simulink model "SystemQ"  (R2014b)
settings: Solver=ode23  StartTime=0.0  StopTime=inf  RelTol=10e-3
PreLoadFcn:
  | initSysQ;
  | runSysQ;
undefined symbols (not defined in the file): Controllers, CR, dim, fdesignblkfcn, G, gcbh, lib, serial, Tjoint, Tpid, X, Y, Z
libraries: sm_lib x62, nesl_utility x28, simulink x10, roblocks x5, instrumentlib x2, dspmathops x1, dspinverses x1, dspmtrx3 x1
(part 3 of 3)

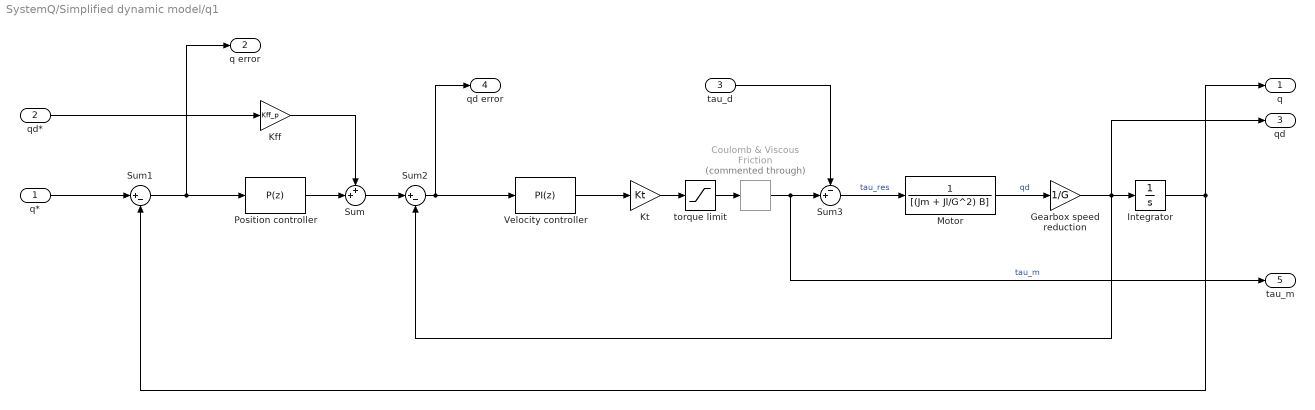
== system SystemQ/Simplified dynamic model/q1 ==
  q* : Inport
  qd* : Inport  Port=2
  tau_d : Inport  Port=3
  Coulomb & Viscous Friction : simulink/Discontinuities/Coulomb & Viscous Friction  Commented=through  offset=0.126  gain=1
  Gearbox speed reduction : Gain  Gain=1/G
  Integrator : Integrator
  Kff : Gain  Gain=Kff_p
  Kt : Gain  Gain=Kt
  Motor : TransferFcn  Denominator=[(Jm + Jl/G^2) B]  ContinuousStateAttributes='qd'
  Position controller : simulink/Continuous/PID Controller  Controller=P  TimeDomain=Discrete-time  SampleTime=Ts  IntegratorMethod=Forward Euler  FilterMethod=Forward Euler  Form=Parallel  P=Kp_p  I=Ki_p  D=Kd_p  N=100  InitialConditionSource=internal  InitialConditionForIntegrator=0  InitialConditionForFilter=0  ExternalReset=none  LimitOutput=off  UpperSaturationLimit=1  LowerSaturationLimit=-1  LinearizeAsGain=on  AntiWindupMode=none  Kb=1  TrackingMode=off  Kt=1  PParamMin=[]  PParamMax=[]  IParamMin=[]  IParamMax=[]  DParamMin=[]  DParamMax=[]  NParamMin=[]  NParamMax=[]  KbParamMin=[]  KbParamMax=[]  KtParamMin=[]  KtParamMax=[]  POutMin=[]  POutMax=[]  IOutMin=[]  IOutMax=[]  DOutMin=[]  DOutMax=[]  NOutMin=[]  NOutMax=[]  KbOutMin=[]  KbOutMax=[]  KtOutMin=[]  KtOutMax=[]  IntegratorOutMin=[]  IntegratorOutMax=[]  FilterOutMin=[]  FilterOutMax=[]  SumOutMin=[]  SumOutMax=[]  SumI1OutMin=[]  SumI1OutMax=[]  SumI2OutMin=[]  SumI2OutMax=[]  SumI3OutMin=[]  SumI3OutMax=[]  SumDOutMin=[]  SumDOutMax=[]  SaturationOutMin=[]  SaturationOutMax=[]  IntegratorContinuousStateAttributes=''  IntegratorStateMustResolveToSignalObject=off  IntegratorRTWStateStorageClass=Auto  FilterContinuousStateAttributes=''  FilterStateMustResolveToSignalObject=off  FilterRTWStateStorageClass=Auto  DifferentiatorICPrevScaledInput=0  DifferentiatorOutMin=[]  DifferentiatorOutMax=[]  UseFilter=on
  Sum : Sum  Inputs=++|
  Sum1 : Sum  Inputs=|+-
  Sum2 : Sum  Inputs=|+-
  Sum3 : Sum  Inputs=-+|
  Velocity controller : simulink/Continuous/PID Controller  Controller=PI  TimeDomain=Discrete-time  SampleTime=Ts  IntegratorMethod=Forward Euler  FilterMethod=Forward Euler  Form=Parallel  P=Kp_v  I=Ki_v  D=Kd_v  N=100  InitialConditionSource=internal  InitialConditionForIntegrator=0  InitialConditionForFilter=0  ExternalReset=none  LimitOutput=on  UpperSaturationLimit=4  LowerSaturationLimit=-4  LinearizeAsGain=on  AntiWindupMode=clamping  Kb=1  TrackingMode=off  Kt=1  PParamMin=[]  PParamMax=[]  IParamMin=[]  IParamMax=[]  DParamMin=[]  DParamMax=[]  NParamMin=[]  NParamMax=[]  KbParamMin=[]  KbParamMax=[]  KtParamMin=[]  KtParamMax=[]  POutMin=[]  POutMax=[]  IOutMin=[]  IOutMax=[]  DOutMin=[]  DOutMax=[]  NOutMin=[]  NOutMax=[]  KbOutMin=[]  KbOutMax=[]  KtOutMin=[]  KtOutMax=[]  IntegratorOutMin=[]  IntegratorOutMax=[]  FilterOutMin=[]  FilterOutMax=[]  SumOutMin=[]  SumOutMax=[]  SumI1OutMin=[]  SumI1OutMax=[]  SumI2OutMin=[]  SumI2OutMax=[]  SumI3OutMin=[]  SumI3OutMax=[]  SumDOutMin=[]  SumDOutMax=[]  SaturationOutMin=[]  SaturationOutMax=[]  IntegratorContinuousStateAttributes=''  IntegratorStateMustResolveToSignalObject=off  IntegratorRTWStateStorageClass=Auto  FilterContinuousStateAttributes=''  FilterStateMustResolveToSignalObject=off  FilterRTWStateStorageClass=Auto  DifferentiatorICPrevScaledInput=0  DifferentiatorOutMin=[]  DifferentiatorOutMax=[]  UseFilter=on
  torque limit : Saturate  UpperLimit=tau_max  LowerLimit=-tau_max
  q : Outport
  q error : Outport  Port=2
  qd : Outport  Port=3
  qd error : Outport  Port=4
  tau_m : Outport  Port=5
  wires:
  Sum1/1 -> Position controller/1, q error/1
  q*/1 -> Sum1/1
  Integrator/1 -> Sum1/2, q/1
  Sum/1 -> Sum2/1
  Sum3/1 -> Motor/1  "tau_res"
  Sum2/1 -> Velocity controller/1, qd error/1
  Motor/1 -> Gearbox speed reduction/1  "qd"
  tau_d/1 -> Sum3/1
  torque limit/1 -> Coulomb & Viscous Friction/1
  qd*/1 -> Kff/1
  Kt/1 -> torque limit/1
  Velocity controller/1 -> Kt/1
  Kff/1 -> Sum/1
  Position controller/1 -> Sum/2
  Coulomb & Viscous Friction/1 -> Sum3/2, tau_m/1  "tau_m"
  Gearbox speed reduction/1 -> Sum2/2, qd/1, Integrator/1

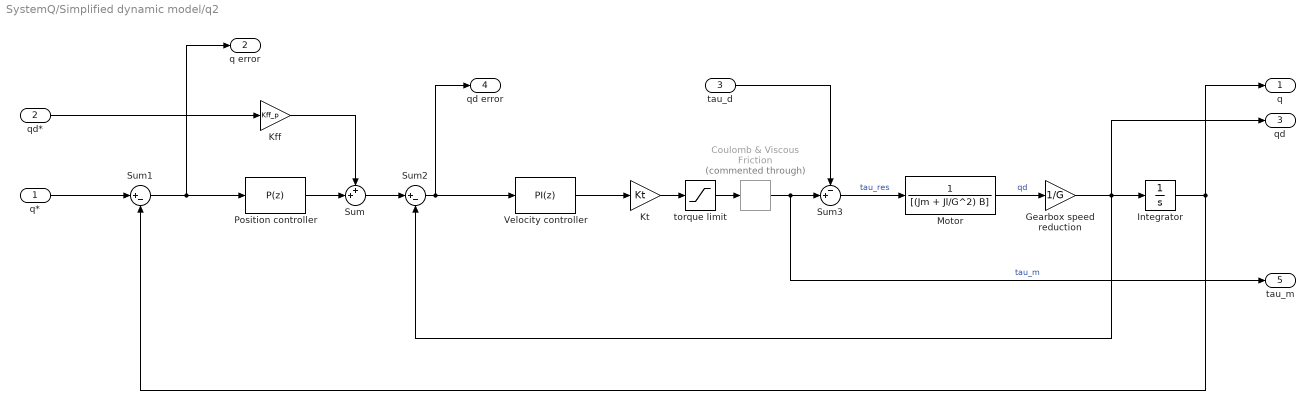
== system SystemQ/Simplified dynamic model/q2 ==
  q* : Inport
  qd* : Inport  Port=2
  tau_d : Inport  Port=3
  Coulomb & Viscous Friction : simulink/Discontinuities/Coulomb & Viscous Friction  Commented=through  offset=0.126  gain=1
  Gearbox speed reduction : Gain  Gain=1/G
  Integrator : Integrator
  Kff : Gain  Gain=Kff_p
  Kt : Gain  Gain=Kt
  Motor : TransferFcn  Denominator=[(Jm + Jl/G^2) B]  ContinuousStateAttributes='qd'
  Position controller : simulink/Continuous/PID Controller  Controller=P  TimeDomain=Discrete-time  SampleTime=Ts  IntegratorMethod=Forward Euler  FilterMethod=Forward Euler  Form=Parallel  P=Kp_p  I=Ki_p  D=Kd_p  N=100  InitialConditionSource=internal  InitialConditionForIntegrator=0  InitialConditionForFilter=0  ExternalReset=none  LimitOutput=off  UpperSaturationLimit=1  LowerSaturationLimit=-1  LinearizeAsGain=on  AntiWindupMode=none  Kb=1  TrackingMode=off  Kt=1  PParamMin=[]  PParamMax=[]  IParamMin=[]  IParamMax=[]  DParamMin=[]  DParamMax=[]  NParamMin=[]  NParamMax=[]  KbParamMin=[]  KbParamMax=[]  KtParamMin=[]  KtParamMax=[]  POutMin=[]  POutMax=[]  IOutMin=[]  IOutMax=[]  DOutMin=[]  DOutMax=[]  NOutMin=[]  NOutMax=[]  KbOutMin=[]  KbOutMax=[]  KtOutMin=[]  KtOutMax=[]  IntegratorOutMin=[]  IntegratorOutMax=[]  FilterOutMin=[]  FilterOutMax=[]  SumOutMin=[]  SumOutMax=[]  SumI1OutMin=[]  SumI1OutMax=[]  SumI2OutMin=[]  SumI2OutMax=[]  SumI3OutMin=[]  SumI3OutMax=[]  SumDOutMin=[]  SumDOutMax=[]  SaturationOutMin=[]  SaturationOutMax=[]  IntegratorContinuousStateAttributes=''  IntegratorStateMustResolveToSignalObject=off  IntegratorRTWStateStorageClass=Auto  FilterContinuousStateAttributes=''  FilterStateMustResolveToSignalObject=off  FilterRTWStateStorageClass=Auto  DifferentiatorICPrevScaledInput=0  DifferentiatorOutMin=[]  DifferentiatorOutMax=[]  UseFilter=on
  Sum : Sum  Inputs=++|
  Sum1 : Sum  Inputs=|+-
  Sum2 : Sum  Inputs=|+-
  Sum3 : Sum  Inputs=-+|
  Velocity controller : simulink/Continuous/PID Controller  Controller=PI  TimeDomain=Discrete-time  SampleTime=Ts  IntegratorMethod=Forward Euler  FilterMethod=Forward Euler  Form=Parallel  P=Kp_v  I=Ki_v  D=Kd_v  N=100  InitialConditionSource=internal  InitialConditionForIntegrator=0  InitialConditionForFilter=0  ExternalReset=none  LimitOutput=on  UpperSaturationLimit=4  LowerSaturationLimit=-4  LinearizeAsGain=on  AntiWindupMode=clamping  Kb=1  TrackingMode=off  Kt=1  PParamMin=[]  PParamMax=[]  IParamMin=[]  IParamMax=[]  DParamMin=[]  DParamMax=[]  NParamMin=[]  NParamMax=[]  KbParamMin=[]  KbParamMax=[]  KtParamMin=[]  KtParamMax=[]  POutMin=[]  POutMax=[]  IOutMin=[]  IOutMax=[]  DOutMin=[]  DOutMax=[]  NOutMin=[]  NOutMax=[]  KbOutMin=[]  KbOutMax=[]  KtOutMin=[]  KtOutMax=[]  IntegratorOutMin=[]  IntegratorOutMax=[]  FilterOutMin=[]  FilterOutMax=[]  SumOutMin=[]  SumOutMax=[]  SumI1OutMin=[]  SumI1OutMax=[]  SumI2OutMin=[]  SumI2OutMax=[]  SumI3OutMin=[]  SumI3OutMax=[]  SumDOutMin=[]  SumDOutMax=[]  SaturationOutMin=[]  SaturationOutMax=[]  IntegratorContinuousStateAttributes=''  IntegratorStateMustResolveToSignalObject=off  IntegratorRTWStateStorageClass=Auto  FilterContinuousStateAttributes=''  FilterStateMustResolveToSignalObject=off  FilterRTWStateStorageClass=Auto  DifferentiatorICPrevScaledInput=0  DifferentiatorOutMin=[]  DifferentiatorOutMax=[]  UseFilter=on
  torque limit : Saturate  UpperLimit=tau_max  LowerLimit=-tau_max
  q : Outport
  q error : Outport  Port=2
  qd : Outport  Port=3
  qd error : Outport  Port=4
  tau_m : Outport  Port=5
  wires:
  Sum1/1 -> Position controller/1, q error/1
  q*/1 -> Sum1/1
  Integrator/1 -> Sum1/2, q/1
  Sum/1 -> Sum2/1
  Sum3/1 -> Motor/1  "tau_res"
  Sum2/1 -> Velocity controller/1, qd error/1
  Motor/1 -> Gearbox speed reduction/1  "qd"
  tau_d/1 -> Sum3/1
  torque limit/1 -> Coulomb & Viscous Friction/1
  qd*/1 -> Kff/1
  Kt/1 -> torque limit/1
  Velocity controller/1 -> Kt/1
  Kff/1 -> Sum/1
  Position controller/1 -> Sum/2
  Coulomb & Viscous Friction/1 -> Sum3/2, tau_m/1  "tau_m"
  Gearbox speed reduction/1 -> Sum2/2, qd/1, Integrator/1

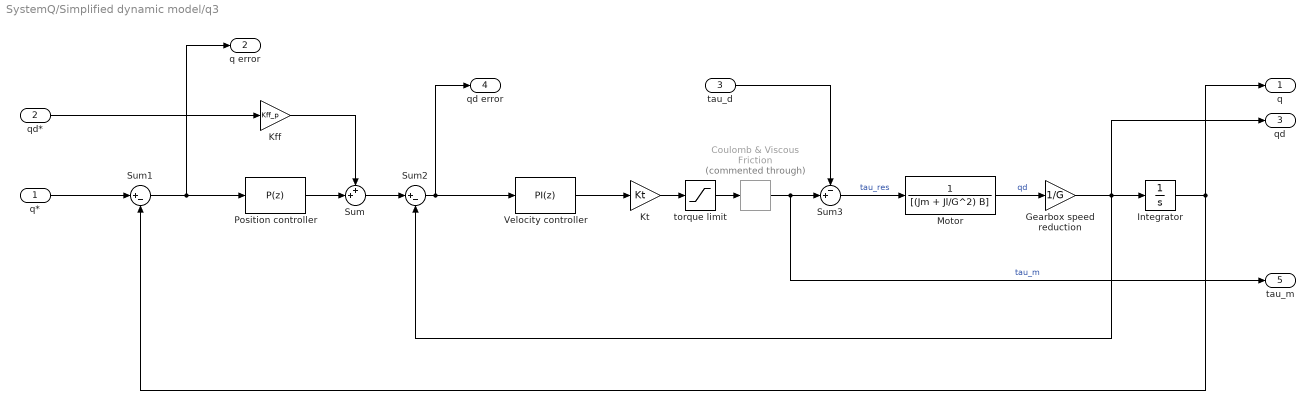
== system SystemQ/Simplified dynamic model/q3 ==
  q* : Inport
  qd* : Inport  Port=2
  tau_d : Inport  Port=3
  Coulomb & Viscous Friction : simulink/Discontinuities/Coulomb & Viscous Friction  Commented=through  offset=0.126  gain=1
  Gearbox speed reduction : Gain  Gain=1/G
  Integrator : Integrator
  Kff : Gain  Gain=Kff_p
  Kt : Gain  Gain=Kt
  Motor : TransferFcn  Denominator=[(Jm + Jl/G^2) B]  ContinuousStateAttributes='qd'
  Position controller : simulink/Continuous/PID Controller  Controller=P  TimeDomain=Discrete-time  SampleTime=Ts  IntegratorMethod=Forward Euler  FilterMethod=Forward Euler  Form=Parallel  P=Kp_p  I=Ki_p  D=Kd_p  N=100  InitialConditionSource=internal  InitialConditionForIntegrator=0  InitialConditionForFilter=0  ExternalReset=none  LimitOutput=off  UpperSaturationLimit=1  LowerSaturationLimit=-1  LinearizeAsGain=on  AntiWindupMode=none  Kb=1  TrackingMode=off  Kt=1  PParamMin=[]  PParamMax=[]  IParamMin=[]  IParamMax=[]  DParamMin=[]  DParamMax=[]  NParamMin=[]  NParamMax=[]  KbParamMin=[]  KbParamMax=[]  KtParamMin=[]  KtParamMax=[]  POutMin=[]  POutMax=[]  IOutMin=[]  IOutMax=[]  DOutMin=[]  DOutMax=[]  NOutMin=[]  NOutMax=[]  KbOutMin=[]  KbOutMax=[]  KtOutMin=[]  KtOutMax=[]  IntegratorOutMin=[]  IntegratorOutMax=[]  FilterOutMin=[]  FilterOutMax=[]  SumOutMin=[]  SumOutMax=[]  SumI1OutMin=[]  SumI1OutMax=[]  SumI2OutMin=[]  SumI2OutMax=[]  SumI3OutMin=[]  SumI3OutMax=[]  SumDOutMin=[]  SumDOutMax=[]  SaturationOutMin=[]  SaturationOutMax=[]  IntegratorContinuousStateAttributes=''  IntegratorStateMustResolveToSignalObject=off  IntegratorRTWStateStorageClass=Auto  FilterContinuousStateAttributes=''  FilterStateMustResolveToSignalObject=off  FilterRTWStateStorageClass=Auto  DifferentiatorICPrevScaledInput=0  DifferentiatorOutMin=[]  DifferentiatorOutMax=[]  UseFilter=on
  Sum : Sum  Inputs=++|
  Sum1 : Sum  Inputs=|+-
  Sum2 : Sum  Inputs=|+-
  Sum3 : Sum  Inputs=-+|
  Velocity controller : simulink/Continuous/PID Controller  Controller=PI  TimeDomain=Discrete-time  SampleTime=Ts  IntegratorMethod=Forward Euler  FilterMethod=Forward Euler  Form=Parallel  P=Kp_v  I=Ki_v  D=Kd_v  N=100  InitialConditionSource=internal  InitialConditionForIntegrator=0  InitialConditionForFilter=0  ExternalReset=none  LimitOutput=on  UpperSaturationLimit=4  LowerSaturationLimit=-4  LinearizeAsGain=on  AntiWindupMode=clamping  Kb=1  TrackingMode=off  Kt=1  PParamMin=[]  PParamMax=[]  IParamMin=[]  IParamMax=[]  DParamMin=[]  DParamMax=[]  NParamMin=[]  NParamMax=[]  KbParamMin=[]  KbParamMax=[]  KtParamMin=[]  KtParamMax=[]  POutMin=[]  POutMax=[]  IOutMin=[]  IOutMax=[]  DOutMin=[]  DOutMax=[]  NOutMin=[]  NOutMax=[]  KbOutMin=[]  KbOutMax=[]  KtOutMin=[]  KtOutMax=[]  IntegratorOutMin=[]  IntegratorOutMax=[]  FilterOutMin=[]  FilterOutMax=[]  SumOutMin=[]  SumOutMax=[]  SumI1OutMin=[]  SumI1OutMax=[]  SumI2OutMin=[]  SumI2OutMax=[]  SumI3OutMin=[]  SumI3OutMax=[]  SumDOutMin=[]  SumDOutMax=[]  SaturationOutMin=[]  SaturationOutMax=[]  IntegratorContinuousStateAttributes=''  IntegratorStateMustResolveToSignalObject=off  IntegratorRTWStateStorageClass=Auto  FilterContinuousStateAttributes=''  FilterStateMustResolveToSignalObject=off  FilterRTWStateStorageClass=Auto  DifferentiatorICPrevScaledInput=0  DifferentiatorOutMin=[]  DifferentiatorOutMax=[]  UseFilter=on
  torque limit : Saturate  UpperLimit=tau_max  LowerLimit=-tau_max
  q : Outport
  q error : Outport  Port=2
  qd : Outport  Port=3
  qd error : Outport  Port=4
  tau_m : Outport  Port=5
  wires:
  Sum1/1 -> Position controller/1, q error/1
  q*/1 -> Sum1/1
  Integrator/1 -> Sum1/2, q/1
  Sum/1 -> Sum2/1
  Sum3/1 -> Motor/1  "tau_res"
  Sum2/1 -> Velocity controller/1, qd error/1
  Motor/1 -> Gearbox speed reduction/1  "qd"
  tau_d/1 -> Sum3/1
  torque limit/1 -> Coulomb & Viscous Friction/1
  qd*/1 -> Kff/1
  Kt/1 -> torque limit/1
  Velocity controller/1 -> Kt/1
  Kff/1 -> Sum/1
  Position controller/1 -> Sum/2
  Coulomb & Viscous Friction/1 -> Sum3/2, tau_m/1  "tau_m"
  Gearbox speed reduction/1 -> Sum2/2, qd/1, Integrator/1

== system SystemQ/Arduino data collecting/Acc. filter/Lowpass Filter ==
  In : Inport
  Generated Filter Block : DiscreteFir  Tag=BlockMethodSubSystem  Coefficients=[0.012742901151903427 -0.056800702054434916 -0.059982833693567543 0.29300036476275532 0.57505703151959175 0.29300036476275532 -0.059982833693567543 -0.056800702054434916 0.012742901151903427]  InputProcessing=Columns as channels (frame based)
  Out : Outport
  wires:
  In/1 -> Generated Filter Block/1
  Generated Filter Block/1 -> Out/1

== system SystemQ/Arduino data collecting/Acc. filter/Lowpass Filter1 ==
  In : Inport
  Generated Filter Block : DiscreteFir  Tag=BlockMethodSubSystem  Coefficients=[0.012742901151903427 -0.056800702054434916 -0.059982833693567543 0.29300036476275532 0.57505703151959175 0.29300036476275532 -0.059982833693567543 -0.056800702054434916 0.012742901151903427]  InputProcessing=Columns as channels (frame based)
  Out : Outport
  wires:
  Generated Filter Block/1 -> Out/1
  In/1 -> Generated Filter Block/1

== system SystemQ/Arduino data collecting/Acc. filter/Lowpass Filter2 ==
  In : Inport
  Generated Filter Block : DiscreteFir  Tag=BlockMethodSubSystem  Coefficients=[0.012742901151903427 -0.056800702054434916 -0.059982833693567543 0.29300036476275532 0.57505703151959175 0.29300036476275532 -0.059982833693567543 -0.056800702054434916 0.012742901151903427]  InputProcessing=Columns as channels (frame based)
  Out : Outport
  wires:
  In/1 -> Generated Filter Block/1
  Generated Filter Block/1 -> Out/1

== stateflow chart SystemQ/Ball release system/BallChart ==
  state RAGGIUNGO/
    status = 0;
  state AGGANCIO/
    status = 1;
  state RILASCIO/
    status = 2;
  (default) -> RAGGIUNGO
  RAGGIUNGO -> AGGANCIO : [error1< 0.05]
  AGGANCIO -> RILASCIO : [error2 < 0.05]
  data: error1 input; error2 input; status output int16
